simulink model "dynamical_model"  (R2023b)
settings: Solver=FixedStepAuto  StartTime=0.0  StopTime=t(end)  FixedStep=0.002  RelTol=1e-3
values from neighbouring files (symbols this model uses):
  beta = kt^2/Rm    [param_id_2dof.m]
  beta_yaw = 0.0051079    [param_id_2dof.m]
  cneg = cneg    [param_id_2dof.m]
  cpos = cQp    [param_id_2dof.m]
  fd = 0.0029    [param_id_2dof.m]
  force_coef = [kTp1, kTp2, kTn1, kTn2]    [param_id_2dof.m]
  fs = 0.0088    [param_id_2dof.m]
  gamma1 = opt_parameters(3)    [param_id_2dof.m]
  I = 1/mu*100    [param_id_2dof.m]
  mu = opt_parameters(1)/(1+opt_parameters(1)*gamma2)    [param_id_2dof.m]
  P = tau*I    [param_id_2dof.m]
  parameters = [Jx1, Jy1, Jz1, Jx2, Jy2, Jz2, beta_pitch, beta_yaw, fs, fd, mode]    [param_id_2dof.m]
  tau = opt_parameters(2)/(1+opt_parameters(1)*gamma2)    [param_id_2dof.m]
undefined symbols (not defined in the file or in its folder): D_position, Dm, Dt, g, Jy, kTn1, kTn2, kTp1, kTp2, Mb, P_position
libraries: slpidlib x2
settings Model: Creator=lmarz  LastModifiedBy=franc
settings RTWCC: GPUComputeCapability=5.0

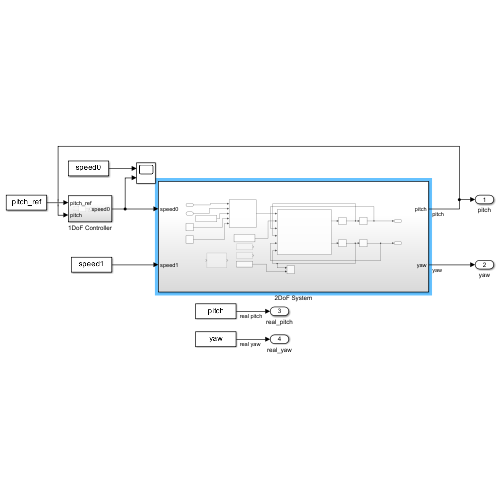
[thumbnail: Simulink's stored preview of the top-level diagram]
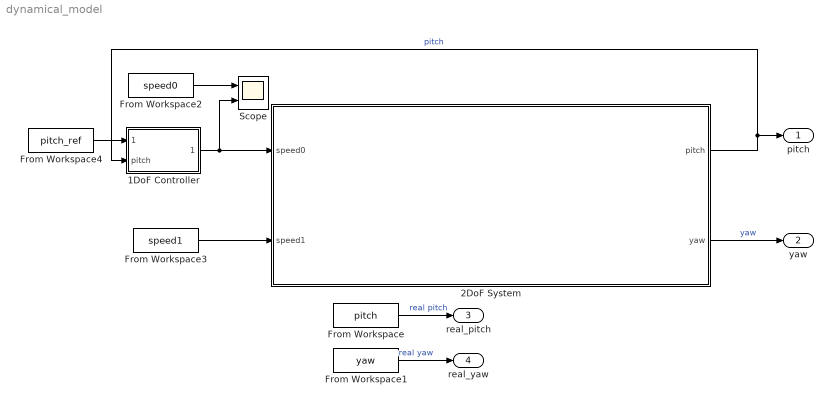
== system dynamical_model ==
  1DoF Controller : Subsystem
  2DoF System : Subsystem
  From Workspace : FromWorkspace  VariableName=pitch  SampleTime=1/500
  From Workspace1 : FromWorkspace  VariableName=yaw  SampleTime=1/500
  From Workspace2 : FromWorkspace  VariableName=speed0  SampleTime=1/500
  From Workspace3 : FromWorkspace  VariableName=speed1  SampleTime=1/500
  From Workspace4 : FromWorkspace  VariableName=pitch_ref  SampleTime=1/500
  Scope : Scope  NumInputPorts=2
  pitch : Outport
  yaw : Outport  Port=2
  real_pitch : Outport  Port=3
  real_yaw : Outport  Port=4
  wires:
  2DoF System/1(pitch) -> 1DoF Controller/2(pitch), pitch/1  "pitch"
  From Workspace1/1 -> real_yaw/1  "real yaw"
  From Workspace3/1 -> 2DoF System/2(speed1)
  From Workspace4/1 -> 1DoF Controller/1(pitch_ref)
  1DoF Controller/1(speed0) -> 2DoF System/1(speed0), Scope/2
  From Workspace2/1 -> Scope/1
  2DoF System/2(yaw) -> yaw/1  "yaw"
  From Workspace/1 -> real_pitch/1  "real pitch"

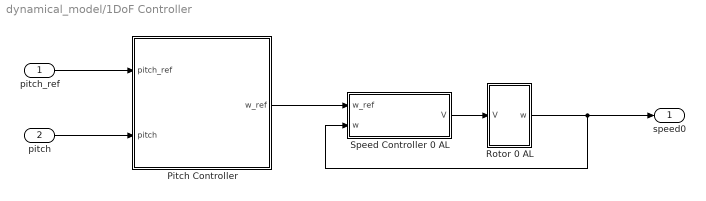
== system dynamical_model/1DoF Controller ==
  pitch_ref : Inport
  pitch : Inport  Port=2
  Pitch Controller : Subsystem
  Rotor 0 AL : Subsystem
  Speed Controller 0 AL : Subsystem
  speed0 : Outport
  wires:
  Speed Controller 0 AL/1(V) -> Rotor 0 AL/1(V)
  Rotor 0 AL/1(w) -> Speed Controller 0 AL/2(w), speed0/1
  Pitch Controller/1(w_ref) -> Speed Controller 0 AL/1(w_ref)
  pitch_ref/1 -> Pitch Controller/1(pitch_ref)
  pitch/1 -> Pitch Controller/2(pitch)

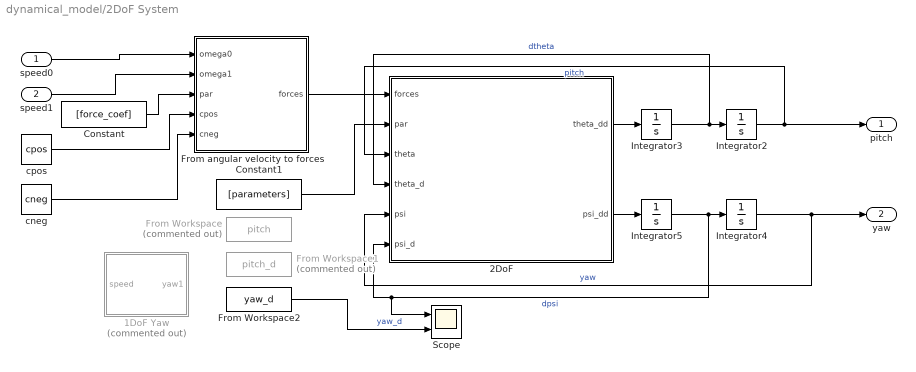
== system dynamical_model/2DoF System ==
  speed0 : Inport
  speed1 : Inport  Port=2
  1DoF Yaw : Subsystem  Commented=on
  2DoF : MATLAB Function  TreatAsAtomicUnit=on
  Constant : Constant  Value=[force_coef]
  Constant1 : Constant  Value=[parameters]
  From Workspace : FromWorkspace  Commented=on  VariableName=pitch  SampleTime=1/500
  From Workspace1 : FromWorkspace  Commented=on  VariableName=pitch_d  SampleTime=1/500
  From Workspace2 : FromWorkspace  VariableName=yaw_d  SampleTime=1/500
  From angular velocity to forces : MATLAB Function  TreatAsAtomicUnit=on
  Integrator{2..5} (4 alike) : Integrator
  Scope : Scope  NumInputPorts=2
  cneg : Constant  Value=cneg
  cpos : Constant  Value=cpos
  pitch : Outport
  yaw : Outport  Port=2
  wires:
  Integrator2/1 -> 2DoF/3(theta), pitch/1  "pitch"
  speed1/1 -> From angular velocity to forces/2(omega1)
  Integrator4/1 -> yaw/1, 2DoF/5(psi)  "yaw"
  speed0/1 -> From angular velocity to forces/1(omega0)
  2DoF/1(theta_dd) -> Integrator3/1
  From angular velocity to forces/1(forces) -> 2DoF/1(forces)
  Integrator3/1 -> Integrator2/1, 2DoF/4(theta_d)  "dtheta"
  2DoF/2(psi_dd) -> Integrator5/1
  Integrator5/1 -> Integrator4/1, Scope/1, 2DoF/6(psi_d)  "dpsi"
  Constant/1 -> From angular velocity to forces/3(par)
  Constant1/1 -> 2DoF/2(par)
  cpos/1 -> From angular velocity to forces/4(cpos)
  cneg/1 -> From angular velocity to forces/5(cneg)
  From Workspace2/1 -> Scope/2  "yaw_d"

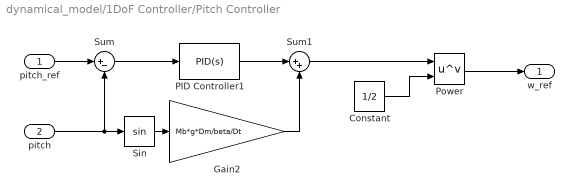
== system dynamical_model/1DoF Controller/Pitch Controller ==
  pitch_ref : Inport
  pitch : Inport  Port=2
  Constant : Constant  Value=1/2
  Gain2 : Gain  Gain=Mb*g*Dm/beta/Dt
  PID Controller1 : slpidlib/PID Controller  Controller=PID  Form=Parallel  TimeDomain=Continuous-time  UseExternalTs=off  SampleTime=1/500  IntegratorMethod=Forward Euler  FilterMethod=Forward Euler  ControllerParametersSource=internal  P=P_position*40  I=5000  UseKiTs=off  D=D_position*5  N=1/0.05  UseFilter=on  TunerSelectOption=Frequency Response Based  InitialConditionSource=internal  InitialConditionForIntegrator=0  InitialConditionForFilter=0  DifferentiatorICPrevScaledInput=0  ExternalReset=none  TrackingMode=off  Kt=1  LimitOutput=on  SatLimitsSource=internal  UpperSaturationLimit=217^2  LowerSaturationLimit=-217^2  LinearizeAsGain=on  AntiWindupMode=clamping  Kb=1  LimitIntegrator=off  UpperIntegratorSaturationLimit=inf  LowerIntegratorSaturationLimit=-inf  POutMin=[]  POutMax=[]  IOutMin=[]  IOutMax=[]  DOutMin=[]  DOutMax=[]  NOutMin=[]  NOutMax=[]  SumOutMin=[]  SumOutMax=[]  SaturationOutMin=[]  SaturationOutMax=[]  PParamMin=[]  PParamMax=[]  IParamMin=[]  IParamMax=[]  DParamMin=[]  DParamMax=[]  NParamMin=[]  NParamMax=[]  KbParamMin=[]  KbParamMax=[]  KtParamMin=[]  KtParamMax=[]  KbOutMin=[]  KbOutMax=[]  KtOutMin=[]  KtOutMax=[]  IntegratorOutMin=[]  IntegratorOutMax=[]  FilterOutMin=[]  FilterOutMax=[]  SumI1OutMin=[]  SumI1OutMax=[]  SumI2OutMin=[]  SumI2OutMax=[]  SumI3OutMin=[]  SumI3OutMax=[]  SumI4OutMin=[]  SumI4OutMax=[]  SumDOutMin=[]  SumDOutMax=[]  DifferentiatorOutMin=[]  DifferentiatorOutMax=[]  FilterDiffOutCoefMin=[]  FilterDiffOutCoefMax=[]  ReciprocalOutMin=[]  ReciprocalOutMax=[]  SumDenOutMin=[]  SumDenOutMax=[]  SumNumOutMin=[]  SumNumOutMax=[]  DivideOutMin=[]  DivideOutMax=[]  UdiffTsProdOutMin=[]  UdiffTsProdOutMax=[]  NTsProdOutMin=[]  NTsProdOutMax=[]  UintegralTsProdOutMin=[]  UintegralTsProdOutMax=[]  UngainTsProdOutMin=[]  UngainTsProdOutMax=[]  ClampingZeroOutDataTypeStr=Inherit: Inherit via back propagation  ClampingZeroOutMin=[]  ClampingZeroOutMax=[]  FilterDenConstantOutDataTypeStr=Inherit: Inherit via back propagation  FilterDenConstantOutMin=[]  FilterDenConstantOutMax=[]  PCopyOutDataTypeStr=Inherit: Inherit via back propagation  PCopyOutMin=[]  PCopyOutMax=[]  NCopyOutDataTypeStr=Inherit: Inherit via back propagation  NCopyOutMin=[]  NCopyOutMax=[]  IntegratorContinuousStateAttributes=''  IntegratorStateMustResolveToSignalObject=off  IntegratorRTWStateStorageClass=Auto  FilterContinuousStateAttributes=''  FilterStateMustResolveToSignalObject=off  FilterRTWStateStorageClass=Auto  ParallelPVariant=InternalParameters  IdealPVariant=Disabled  IVariant=InternalParameters  DVariant=InternalParameters  IntegratorVariant=Continuous  SatVariant=Enabled  AWVariant=ContClampingParallel  PCopyVariant=Disabled  TRVariant=Disabled  FdbkBlocksVariant=Forward  IdealPFdbkVariant=Disabled  SatFdbkVariant=Disabled  DerivativeFilterVariant=ContFilter  NVariant=InternalParameters  NCopyVariant=Disabled  FilterICVariant=InternalICsFilter  IntegratorICVariant=InternalICs  ExternalResetVariant=Disabled  TRSumVariant=Passthrough  SumFdbkVariant=Disabled  SumVariant=Sum_PID  TsampFilterVariant=InternalTs  TsampNgainVariant=Passthrough  TsampIntegralVariant=Disabled_SignalSpec  ExternalSaturationOutDataTypeStr=Inherit: Same as second input
  Power : Math  Operator=pow  SignedPower=on
  Sin : Trigonometry
  Sum : Sum  Inputs=|+-
  Sum1 : Sum  Inputs=|++
  w_ref : Outport
  wires:
  pitch_ref/1 -> Sum/1
  pitch/1 -> Sum/2, Sin/1
  Gain2/1 -> Sum1/2
  Sum/1 -> PID Controller1/1
  Sin/1 -> Gain2/1
  PID Controller1/1 -> Sum1/1
  Sum1/1 -> Power/1
  Power/1 -> w_ref/1
  Constant/1 -> Power/2

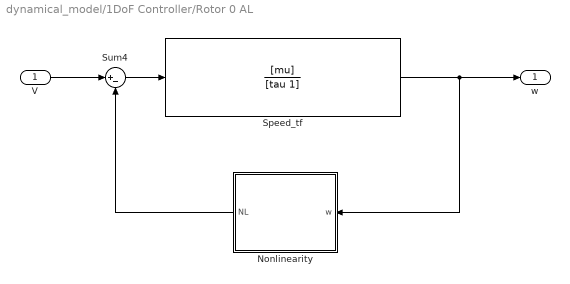
== system dynamical_model/1DoF Controller/Rotor 0 AL ==
  V : Inport
  Nonlinearity : Subsystem
  Speed_tf : TransferFcn  Numerator=[mu]  Denominator=[tau 1]
  Sum4 : Sum  Inputs=|+-
  w : Outport
  wires:
  V/1 -> Sum4/1
  Sum4/1 -> Speed_tf/1
  Speed_tf/1 -> Nonlinearity/1(w), w/1
  Nonlinearity/1(NL) -> Sum4/2

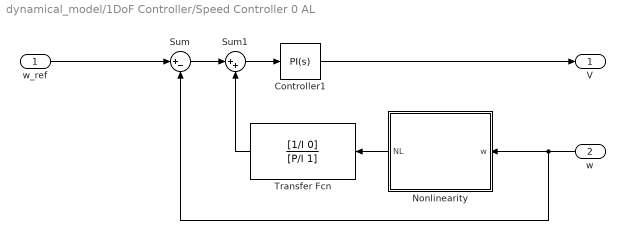
== system dynamical_model/1DoF Controller/Speed Controller 0 AL ==
  w_ref : Inport
  w : Inport  Port=2
  Controller1 : slpidlib/PID Controller  Controller=PI  Form=Parallel  TimeDomain=Continuous-time  UseExternalTs=off  SampleTime=-1  IntegratorMethod=Forward Euler  FilterMethod=Forward Euler  ControllerParametersSource=internal  P=P  I=I  UseKiTs=off  D=0  N=100  UseFilter=on  TunerSelectOption=Transfer Function Based (PID Tuner App)  InitialConditionSource=internal  InitialConditionForIntegrator=0  InitialConditionForFilter=0  DifferentiatorICPrevScaledInput=0  ExternalReset=none  TrackingMode=off  Kt=1  LimitOutput=on  SatLimitsSource=internal  UpperSaturationLimit=18  LowerSaturationLimit=-18  LinearizeAsGain=off  AntiWindupMode=clamping  Kb=1  LimitIntegrator=off  UpperIntegratorSaturationLimit=inf  LowerIntegratorSaturationLimit=-inf  POutMin=[]  POutMax=[]  IOutMin=[]  IOutMax=[]  DOutMin=[]  DOutMax=[]  NOutMin=[]  NOutMax=[]  SumOutMin=[]  SumOutMax=[]  SaturationOutMin=[]  SaturationOutMax=[]  PParamMin=[]  PParamMax=[]  IParamMin=[]  IParamMax=[]  DParamMin=[]  DParamMax=[]  NParamMin=[]  NParamMax=[]  KbParamMin=[]  KbParamMax=[]  KtParamMin=[]  KtParamMax=[]  KbOutMin=[]  KbOutMax=[]  KtOutMin=[]  KtOutMax=[]  IntegratorOutMin=[]  IntegratorOutMax=[]  FilterOutMin=[]  FilterOutMax=[]  SumI1OutMin=[]  SumI1OutMax=[]  SumI2OutMin=[]  SumI2OutMax=[]  SumI3OutMin=[]  SumI3OutMax=[]  SumI4OutMin=[]  SumI4OutMax=[]  SumDOutMin=[]  SumDOutMax=[]  DifferentiatorOutMin=[]  DifferentiatorOutMax=[]  FilterDiffOutCoefMin=[]  FilterDiffOutCoefMax=[]  ReciprocalOutMin=[]  ReciprocalOutMax=[]  SumDenOutMin=[]  SumDenOutMax=[]  SumNumOutMin=[]  SumNumOutMax=[]  DivideOutMin=[]  DivideOutMax=[]  UdiffTsProdOutMin=[]  UdiffTsProdOutMax=[]  NTsProdOutMin=[]  NTsProdOutMax=[]  UintegralTsProdOutMin=[]  UintegralTsProdOutMax=[]  UngainTsProdOutMin=[]  UngainTsProdOutMax=[]  ClampingZeroOutDataTypeStr=Inherit: Inherit via back propagation  ClampingZeroOutMin=[]  ClampingZeroOutMax=[]  FilterDenConstantOutDataTypeStr=Inherit: Inherit via back propagation  FilterDenConstantOutMin=[]  FilterDenConstantOutMax=[]  PCopyOutDataTypeStr=Inherit: Inherit via back propagation  PCopyOutMin=[]  PCopyOutMax=[]  NCopyOutDataTypeStr=Inherit: Inherit via back propagation  NCopyOutMin=[]  NCopyOutMax=[]  IntegratorContinuousStateAttributes=''  IntegratorStateMustResolveToSignalObject=off  IntegratorRTWStateStorageClass=Auto  FilterContinuousStateAttributes=''  FilterStateMustResolveToSignalObject=off  FilterRTWStateStorageClass=Auto  ParallelPVariant=InternalParameters  IdealPVariant=Disabled  IVariant=InternalParameters  DVariant=Disabled  IntegratorVariant=Continuous  SatVariant=Enabled  AWVariant=ContClampingParallel  PCopyVariant=Disabled  TRVariant=Disabled  FdbkBlocksVariant=Forward  IdealPFdbkVariant=Disabled  SatFdbkVariant=Disabled  DerivativeFilterVariant=Disabled  NVariant=Disabled  NCopyVariant=Disabled_SignalSpec  FilterICVariant=Disabled  IntegratorICVariant=InternalICs  ExternalResetVariant=Disabled  TRSumVariant=Passthrough  SumFdbkVariant=Disabled  SumVariant=Sum_PI  TsampFilterVariant=InternalTs  TsampNgainVariant=Passthrough  TsampIntegralVariant=Disabled_SignalSpec  ExternalSaturationOutDataTypeStr=Inherit: Same as second input
  Nonlinearity : Subsystem
  Sum : Sum  Inputs=|+-
  Sum1 : Sum  Inputs=|++
  Transfer Fcn : TransferFcn  Numerator=[1/I 0]  Denominator=[P/I 1]
  V : Outport
  wires:
  w/1 -> Sum/2, Nonlinearity/1(w)
  w_ref/1 -> Sum/1
  Controller1/1 -> V/1
  Sum1/1 -> Controller1/1
  Nonlinearity/1(NL) -> Transfer Fcn/1
  Transfer Fcn/1 -> Sum1/2
  Sum/1 -> Sum1/1

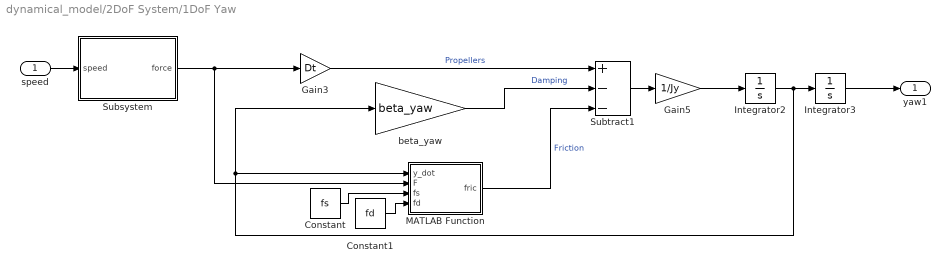
== system dynamical_model/2DoF System/1DoF Yaw ==
  speed : Inport
  Constant : Constant  Value=fs
  Constant1 : Constant  Value=fd
  Gain3 : Gain  Gain=Dt
  Gain5 : Gain  Gain=1/Jy
  Integrator2 : Integrator
  Integrator3 : Integrator
  MATLAB Function : MATLAB Function  TreatAsAtomicUnit=on
  Subsystem : Subsystem
  Subtract1 : Sum  Inputs=+--
  beta_yaw : Gain  Gain=beta_yaw
  yaw1 : Outport
  wires:
  Integrator3/1 -> yaw1/1
  Subtract1/1 -> Gain5/1
  Gain5/1 -> Integrator2/1
  Integrator2/1 -> Integrator3/1, beta_yaw/1, MATLAB Function/1(y_dot)
  MATLAB Function/1(fric) -> Subtract1/3  "Friction"
  beta_yaw/1 -> Subtract1/2  "Damping"
  Gain3/1 -> Subtract1/1  "Propellers"
  Constant/1 -> MATLAB Function/3(fs)
  Constant1/1 -> MATLAB Function/4(fd)
  Subsystem/1(force) -> Gain3/1, MATLAB Function/2(F)
  speed/1 -> Subsystem/1(speed)

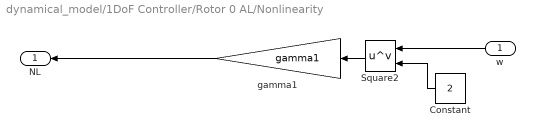
== system dynamical_model/1DoF Controller/Rotor 0 AL/Nonlinearity ==
  w : Inport
  Constant : Constant  Value=2
  Square2 : Math  Operator=pow  SignedPower=on
  gamma1 : Gain  Gain=gamma1
  NL : Outport
  wires:
  Square2/1 -> gamma1/1
  w/1 -> Square2/1
  gamma1/1 -> NL/1
  Constant/1 -> Square2/2

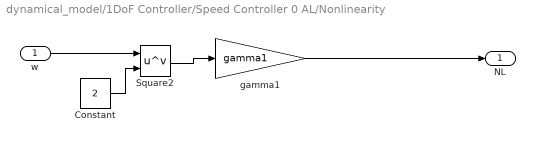
== system dynamical_model/1DoF Controller/Speed Controller 0 AL/Nonlinearity ==
  w : Inport
  Constant : Constant  Value=2
  Square2 : Math  Operator=pow  SignedPower=on
  gamma1 : Gain  Gain=gamma1
  NL : Outport
  wires:
  Square2/1 -> gamma1/1
  w/1 -> Square2/1
  gamma1/1 -> NL/1
  Constant/1 -> Square2/2

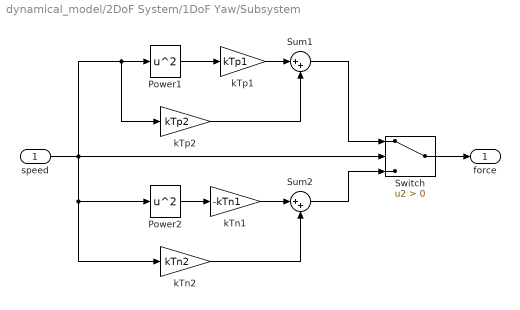
== system dynamical_model/2DoF System/1DoF Yaw/Subsystem ==
  speed : Inport
  Power1 : Math  Operator=square  SignedPower=on
  Power2 : Math  Operator=square  SignedPower=on
  Sum1 : Sum  Inputs=|++
  Sum2 : Sum  Inputs=|++
  Switch : Switch  Criteria=u2 > Threshold  SaturateOnIntegerOverflow=off  InputSameDT=off
  kTn1 : Gain  Gain=-kTn1
  kTn2 : Gain  Gain=kTn2
  kTp1 : Gain  Gain=kTp1
  kTp2 : Gain  Gain=kTp2
  force : Outport
  wires:
  kTp1/1 -> Sum1/1
  speed/1 -> Switch/2, kTn2/1, Power2/1, Power1/1, kTp2/1
  kTn2/1 -> Sum2/2
  Power2/1 -> kTn1/1
  Sum2/1 -> Switch/3
  Power1/1 -> kTp1/1
  kTn1/1 -> Sum2/1
  kTp2/1 -> Sum1/2
  Sum1/1 -> Switch/1
  Switch/1 -> force/1

== matlab function dynamical_model/2DoF System/1DoF Yaw/MATLAB Function ==
  data: y_dot input; fric output; F input; fs input; fd input
function fric = fcn(y_dot, F, fs, fd)

fric  = abs(F);
if fric > fs || y_dot ~= 0
    fric = fd;
end

fric = fric*sign(y_dot);

== matlab function dynamical_model/2DoF System/2DoF ==
  data: forces input; par input; theta input; theta_d input; psi input; psi_d input; theta_dd output; psi_dd output
function [theta_dd, psi_dd]  = model_2dof(forces, par, theta, theta_d, psi, psi_d)%, real_pitch, real_pitch_d, real_yaw_d)

% Assumed to be known parameters
Mb = 1.07; % mass of the upper body
d = 0.0024; % missalignment of the c.o.m. of the upper body
Dt = 0.167; % distance between yaw axis of rotation to motor axis
g = 9.81;

%used in Pitch EoM
yaw_d = psi_d;
% yaw_d = real_yaw_d;

% used in Yaw EoM
pitch = theta;
pitch_d = theta_d;
% pitch = real_pitch;
% pitch_d = real_pitch_d;

% Forces applied 
F0 = forces(1);
F1 = forces(2);
Q0 = forces(3);
Q1 = forces(4);

% Inertia of lower body w.r.t. its local reference frame.
Jx1 = par(1);
Jy1 = par(2);
Jz1 = par(3);

% Inertial of upper body w.r.t its local reference frame.
Jx2 = par(4);
Jy2 = par(5);
Jz2 = par(6);

beta_pitch = par(7); % Damping due to yaw rotation
beta_yaw = par(8); % Damping due to pitch rotation

fs = par(9);
fd = par(10);

mode = par(11);

% Coefficents multiplied by theta_dot_dot
J_theta = Jy2 + Mb*d^2;
% Coefficents multiplied by psi_dot_dot
J_psi = Jz1 + Jx2*sin(pitch)^2 + Jz2*cos(pitch)^2 + Mb*d^2*sin(pitch)^2;
% J_psi = Jz1+Jz2; % for 1 DoF Yaw

switch mode
    case 0
        tau_pitch = (F0-F1)*Dt;
        tau_yaw = 0;
    case 1
        tau_pitch = 0;
        tau_yaw = (F0+F1)*Dt*cos(pitch);
    otherwise
        tau_pitch = F0*Dt-Q1;
        % tau_pitch = F0*Dt; % for 1 DoF Pitch
        tau_yaw = (F1*Dt+Q0)*cos(pitch);
        % tau_yaw = (F1*Dt); % for 1 DoF Yaw
end

% Yaw Friction
fric  = abs(tau_yaw);
if fric > fs || abs(psi_d) > 1
    fric = fd;
end
fric = fric*sign(psi_d); % as the friction force is always oppostite to the movement

coupling_term_pitch = -0.5*(Jx2-Jz2+Mb*d^2)*sin(2*theta)*yaw_d^2;
% coupling_term_pitch = 0; % for 1 DoF Pitch
theta_dd = (tau_pitch - beta_pitch*theta_d - coupling_term_pitch - Mb*g*d*sin(theta))/J_theta;

coupling_term_yaw = (Jx2-Jz2+Mb*d^2)*sin(2*pitch)*psi_d*pitch_d;
% coupling_term_yaw = 0; % for 1 DoF Yaw
psi_dd = (tau_yaw - beta_yaw*psi_d - coupling_term_yaw - fric)/J_psi;

== matlab function dynamical_model/2DoF System/From angular velocity to forces ==
  data: omega0 input; forces output; omega1 input; par input; cpos input; cneg input
function forces = fcn(omega0, omega1, par, cpos, cneg)

kTp1 = par(1);
kTp2 = par(2);

kTn1 = par(3);
kTn2 = par(4);

cQ0 = cpos;
cQ1 = cpos;

cQ0n = cneg;
cQ1n = cneg;

if omega0 > 0
    F0 = kTp1*omega0^2 + kTp2*omega0;
    Q0 = 1.5*cQ0*omega0^2;
else
    F0 = (-kTn1*omega0^2 + kTn2*omega0);
    Q0 = -0.5*cQ0n*omega0^2;
end

if omega1 > 0
    F1 = kTp1*omega1^2 + kTp2*omega1;
    Q1 = cQ1*omega1^2;
else
    F1 = 0.05*(-kTn1*omega1^2 + kTn2*omega1);
    Q1 = -0.5*cQ1n*omega1^2;
end

forces = [F0,F1,Q0,Q1];

end
